simulink model "fusionAlg"  (R2018b)
settings: Solver=FixedStepDiscrete  StartTime=0.0  StopTime=inf  FixedStep=0.01  RelTol=1e-3
PostLoadFcn:
  | if any(exist('dsrtsu_mdlpostloadfcn', 'file') ~= 0), dsrtsu_mdlpostloadfcn('Execute', bdroot); end
model workspace (MAT data in the model file):
  handle : class17 (value not decoded)
(part 22 of 24)

== system fusionAlg/FUSION /FUS_DataAdapter/VisionAdapter/ObjAdapter/Obj_31/Subsystem ==
  <OBJ_Lat_Distance> : Inport
  <OBJ_Lat_Distance_STD> : Inport  Port=2
  <OBJ_Long_Distance> : Inport  Port=3
  <OBJ_Long_Distance_STD> : Inport  Port=4
  Bus Creator : BusCreator  Inputs=4  OutDataTypeStr=Bus: FUS_VISION_OBJ_COORD_ST
      settings: InheritFromInputs=off
  Obj_01_coordinate : Outport
  wires:
  <OBJ_Long_Distance>/1 -> Bus Creator/3
  <OBJ_Lat_Distance>/1 -> Bus Creator/1
  <OBJ_Lat_Distance_STD>/1 -> Bus Creator/2
  Bus Creator/1 -> Obj_01_coordinate/1
  <OBJ_Long_Distance_STD>/1 -> Bus Creator/4

== system fusionAlg/FUSION /FUS_DataAdapter/VisionAdapter/ObjAdapter/Obj_31/Subsystem1 ==
  <OBJ_Abs_Long_Velocity> : Inport
  <OBJ_Abs_Long_Velocity_STD> : Inport  Port=2
  <OBJ_Abs_Lat_Velocity> : Inport  Port=3
  <OBJ_Abs_Lat_Velocity_STD> : Inport  Port=4
  Bus Creator : BusCreator  Inputs=4  OutDataTypeStr=Bus: FUS_VISION_OBJ_VELOCITY
      settings: InheritFromInputs=off
  Out1 : Outport
  wires:
  <OBJ_Abs_Lat_Velocity_STD>/1 -> Bus Creator/4
  <OBJ_Abs_Long_Velocity>/1 -> Bus Creator/1
  <OBJ_Abs_Lat_Velocity>/1 -> Bus Creator/3
  <OBJ_Abs_Long_Velocity_STD>/1 -> Bus Creator/2
  Bus Creator/1 -> Out1/1

== system fusionAlg/FUSION /FUS_DataAdapter/VisionAdapter/ObjAdapter/Obj_31/Subsystem2 ==
  <OBJ_Angle_Mid> : Inport
  <OBJ_Angle_Mid_STD> : Inport  Port=2
  Bus Creator : BusCreator  Inputs=2  OutDataTypeStr=Bus: FUS_VISION_OBJ_ANGLE_ST
      settings: InheritFromInputs=off
  Out1 : Outport
  wires:
  <OBJ_Angle_Mid>/1 -> Bus Creator/1
  Bus Creator/1 -> Out1/1
  <OBJ_Angle_Mid_STD>/1 -> Bus Creator/2

== system fusionAlg/FUSION /FUS_DataAdapter/VisionAdapter/ObjAdapter/Obj_31/Subsystem3 ==
  <OBJ_Abs_Long_Acc> : Inport
  <OBJ_Abs_Long_Acc_STD> : Inport  Port=2
  <OBJ_Abs_Lat_Acc> : Inport  Port=3
  <OBJ_Abs_Lat_Acc_STD> : Inport  Port=4
  Bus Creator : BusCreator  Inputs=4  OutDataTypeStr=Bus: FUS_VISION_OBJ_ACCE_ST
      settings: InheritFromInputs=off
  Out1 : Outport
  wires:
  <OBJ_Abs_Long_Acc_STD>/1 -> Bus Creator/2
  <OBJ_Abs_Long_Acc>/1 -> Bus Creator/1
  Bus Creator/1 -> Out1/1
  <OBJ_Abs_Lat_Acc_STD>/1 -> Bus Creator/4
  <OBJ_Abs_Lat_Acc>/1 -> Bus Creator/3

== system fusionAlg/FUSION /FUS_DataAdapter/VisionAdapter/ObjAdapter/Obj_31/Subsystem4 ==
  <OBJ_Length> : Inport
  <OBJ_Width> : Inport  Port=2
  <OBJ_Height> : Inport  Port=3
  Bus Creator : BusCreator  Inputs=3  OutDataTypeStr=Bus: FUS_VISION_BOXSIZE_ST
      settings: InheritFromInputs=off
  Out1 : Outport
  wires:
  Bus Creator/1 -> Out1/1
  <OBJ_Height>/1 -> Bus Creator/3
  <OBJ_Width>/1 -> Bus Creator/2
  <OBJ_Length>/1 -> Bus Creator/1

== system fusionAlg/FUSION /FUS_DataAdapter/VisionAdapter/ObjAdapter/Obj_31/Subsystem5 ==
  Bus Creator : BusCreator  Inputs=3  OutDataTypeStr=Bus: FUS_VISOBJ_UINT8_RESERVED_ST
      settings: InheritFromInputs=off
  Constant1 : Constant  Value=0  OutDataTypeStr=uint8
  Constant2 : Constant  Value=0  OutDataTypeStr=uint8
  Constant3 : Constant  Value=0  OutDataTypeStr=uint8
  reserved1 : Outport
  wires:
  Bus Creator/1 -> reserved1/1
  Constant2/1 -> Bus Creator/1
  Constant1/1 -> Bus Creator/2
  Constant3/1 -> Bus Creator/3

== system fusionAlg/FUSION /FUS_DataAdapter/VisionAdapter/ObjAdapter/Obj_31/Subsystem6 ==
  Bus Creator : BusCreator  Inputs=2  OutDataTypeStr=Bus: FUS_VISOBJ_UINT32_RESERVED_ST
      settings: InheritFromInputs=off
  Constant5 : Constant  Value=0  OutDataTypeStr=uint32
  Constant6 : Constant  Value=0  OutDataTypeStr=uint32
  reserved2 : Outport
  wires:
  Constant5/1 -> Bus Creator/1
  Bus Creator/1 -> reserved2/1
  Constant6/1 -> Bus Creator/2

== system fusionAlg/FUSION /FUS_DataAdapter/VisionAdapter/ObjAdapter/Obj_31/Subsystem7 ==
  note: Fusion
  note: 0 : (BIT_0)Old or New
  note: EyeQ4
  note: 1 : (BIT_1)Predicted or Measured
  note: 2 : (BIT_2)Not Valid or Valid
  note: 0 : Initialized
  note: 1 : Measured
  note: 2 : Predicted
  <OBJ_Measuring_Status> : Inport
  1-D Lookup Table : Lookup_n-D  NumberOfTableDimensions=1  BreakpointsForDimension1=[0,1,2,3,4,5,6,7]  IndexSearchMethod=Linear search  Table=[2,0,1,1,0,0,1,1]  InterpMethod=Flat  InternalRulePriority=Speed  RndMeth=Simplest  InputSameDT=on
  Data Type Conversion1 : DataTypeConversion  OutDataTypeStr=uint32
  Obj_Status : Outport
  wires:
  Data Type Conversion1/1 -> Obj_Status/1  "Obj_Status"
  <OBJ_Measuring_Status>/1 -> 1-D Lookup Table/1
  1-D Lookup Table/1 -> Data Type Conversion1/1  "Obj_Status"

== system fusionAlg/FUSION /FUS_DataAdapter/VisionAdapter/ObjAdapter/Obj_31/Subsystem8 ==
  note: 2 : Truck
  note: 1 : Pedestrian
  note: 2 : Vehicle
  note: 0 : Unfilled
  note: EyeQ4
  note: Fusion
  note: 0 : Unknown
  note: 1 : CAR
  note: 3 : Motorbike
  note: 4 : Bicycle
  note: 5 : Pedestrian
  note: 6 : General_Object
  note: 7 : Animal
  note: 8 : Uncertain_Vcl
  note: 3 : Truck
  note: 4: MoTor bike
  note: 5 : Bicycle
  note: 6 : General object
  note: 7 : Animal
  <OBJ_Object_Class> : Inport
  1-D Lookup Table : Lookup_n-D  NumberOfTableDimensions=1  BreakpointsForDimension1=[0,1,2,3,4,5,6,7,8]  IndexSearchMethod=Linear search  Table=[0,2,3,4,5,1,6,7,0]  InterpMethod=Flat  InternalRulePriority=Speed  RndMeth=Simplest  InputSameDT=on
  Data Type Conversion2 : DataTypeConversion  OutDataTypeStr=uint32
  Obj_Type : Outport
  wires:
  1-D Lookup Table/1 -> Data Type Conversion2/1  "Obj_Status"
  <OBJ_Object_Class>/1 -> 1-D Lookup Table/1
  Data Type Conversion2/1 -> Obj_Type/1  "Obj_Type"

== system fusionAlg/FUSION /FUS_DataAdapter/VisionAdapter/ObjAdapter/Obj_32/Obj_01_Agge ==
  <OBJ_Object_Age> : Inport
  Bus Creator : BusCreator  Inputs=4  OutDataTypeStr=Bus: FUS_VISION_OBJ_STAGE_AGE_ST
      settings: InheritFromInputs=off
  Constant : Constant  Value=3  OutDataTypeStr=uint16
  Constant1 : Constant  Value=2  OutDataTypeStr=uint16
  Data Type Conversion : DataTypeConversion  OutDataTypeStr=uint16
  Obj_01_Age : Outport  OutDataTypeStr=Bus: FUS_VISION_OBJ_STAGE_AGE_ST
  wires:
  Bus Creator/1 -> Obj_01_Age/1
  Constant/1 -> Bus Creator/2
  <OBJ_Object_Age>/1 -> Data Type Conversion/1
  Constant1/1 -> Bus Creator/4
  Data Type Conversion/1 -> Bus Creator/3, Bus Creator/1  "measureAge"

== system fusionAlg/FUSION /FUS_DataAdapter/VisionAdapter/ObjAdapter/Obj_32/Obj_01_boundarhy ==
  Bus Creator : BusCreator  Inputs=4  OutDataTypeStr=Bus: FUS_VISION_OBJ_BOUNDARY
      settings: InheritFromInputs=off
  Constant{,1..3} (4 alike) : Constant  Value=0  OutDataTypeStr=int16
  Obj_01_boundary : Outport  OutDataTypeStr=Bus: FUS_VISION_OBJ_BOUNDARY
  wires:
  Bus Creator/1 -> Obj_01_boundary/1
  Constant/1 -> Bus Creator/1
  Constant1/1 -> Bus Creator/2
  Constant2/1 -> Bus Creator/3
  Constant3/1 -> Bus Creator/4

== system fusionAlg/FUSION /FUS_DataAdapter/VisionAdapter/ObjAdapter/Obj_32/Subsystem ==
  <OBJ_Lat_Distance> : Inport
  <OBJ_Lat_Distance_STD> : Inport  Port=2
  <OBJ_Long_Distance> : Inport  Port=3
  <OBJ_Long_Distance_STD> : Inport  Port=4
  Bus Creator : BusCreator  Inputs=4  OutDataTypeStr=Bus: FUS_VISION_OBJ_COORD_ST
      settings: InheritFromInputs=off
  Obj_01_coordinate : Outport
  wires:
  <OBJ_Long_Distance>/1 -> Bus Creator/3
  <OBJ_Lat_Distance>/1 -> Bus Creator/1
  <OBJ_Lat_Distance_STD>/1 -> Bus Creator/2
  Bus Creator/1 -> Obj_01_coordinate/1
  <OBJ_Long_Distance_STD>/1 -> Bus Creator/4

== system fusionAlg/FUSION /FUS_DataAdapter/VisionAdapter/ObjAdapter/Obj_32/Subsystem1 ==
  <OBJ_Abs_Long_Velocity> : Inport
  <OBJ_Abs_Long_Velocity_STD> : Inport  Port=2
  <OBJ_Abs_Lat_Velocity> : Inport  Port=3
  <OBJ_Abs_Lat_Velocity_STD> : Inport  Port=4
  Bus Creator : BusCreator  Inputs=4  OutDataTypeStr=Bus: FUS_VISION_OBJ_VELOCITY
      settings: InheritFromInputs=off
  Out1 : Outport
  wires:
  <OBJ_Abs_Lat_Velocity_STD>/1 -> Bus Creator/4
  <OBJ_Abs_Long_Velocity>/1 -> Bus Creator/1
  <OBJ_Abs_Lat_Velocity>/1 -> Bus Creator/3
  <OBJ_Abs_Long_Velocity_STD>/1 -> Bus Creator/2
  Bus Creator/1 -> Out1/1

== system fusionAlg/FUSION /FUS_DataAdapter/VisionAdapter/ObjAdapter/Obj_32/Subsystem2 ==
  <OBJ_Angle_Mid> : Inport
  <OBJ_Angle_Mid_STD> : Inport  Port=2
  Bus Creator : BusCreator  Inputs=2  OutDataTypeStr=Bus: FUS_VISION_OBJ_ANGLE_ST
      settings: InheritFromInputs=off
  Out1 : Outport
  wires:
  <OBJ_Angle_Mid>/1 -> Bus Creator/1
  Bus Creator/1 -> Out1/1
  <OBJ_Angle_Mid_STD>/1 -> Bus Creator/2

== system fusionAlg/FUSION /FUS_DataAdapter/VisionAdapter/ObjAdapter/Obj_32/Subsystem3 ==
  <OBJ_Abs_Long_Acc> : Inport
  <OBJ_Abs_Long_Acc_STD> : Inport  Port=2
  <OBJ_Abs_Lat_Acc> : Inport  Port=3
  <OBJ_Abs_Lat_Acc_STD> : Inport  Port=4
  Bus Creator : BusCreator  Inputs=4  OutDataTypeStr=Bus: FUS_VISION_OBJ_ACCE_ST
      settings: InheritFromInputs=off
  Out1 : Outport
  wires:
  <OBJ_Abs_Long_Acc_STD>/1 -> Bus Creator/2
  <OBJ_Abs_Long_Acc>/1 -> Bus Creator/1
  Bus Creator/1 -> Out1/1
  <OBJ_Abs_Lat_Acc_STD>/1 -> Bus Creator/4
  <OBJ_Abs_Lat_Acc>/1 -> Bus Creator/3

== system fusionAlg/FUSION /FUS_DataAdapter/VisionAdapter/ObjAdapter/Obj_32/Subsystem4 ==
  <OBJ_Length> : Inport
  <OBJ_Width> : Inport  Port=2
  <OBJ_Height> : Inport  Port=3
  Bus Creator : BusCreator  Inputs=3  OutDataTypeStr=Bus: FUS_VISION_BOXSIZE_ST
      settings: InheritFromInputs=off
  Out1 : Outport
  wires:
  Bus Creator/1 -> Out1/1
  <OBJ_Height>/1 -> Bus Creator/3
  <OBJ_Width>/1 -> Bus Creator/2
  <OBJ_Length>/1 -> Bus Creator/1

== system fusionAlg/FUSION /FUS_DataAdapter/VisionAdapter/ObjAdapter/Obj_32/Subsystem5 ==
  Bus Creator : BusCreator  Inputs=3  OutDataTypeStr=Bus: FUS_VISOBJ_UINT8_RESERVED_ST
      settings: InheritFromInputs=off
  Constant1 : Constant  Value=0  OutDataTypeStr=uint8
  Constant2 : Constant  Value=0  OutDataTypeStr=uint8
  Constant3 : Constant  Value=0  OutDataTypeStr=uint8
  reserved1 : Outport
  wires:
  Bus Creator/1 -> reserved1/1
  Constant2/1 -> Bus Creator/1
  Constant1/1 -> Bus Creator/2
  Constant3/1 -> Bus Creator/3

== system fusionAlg/FUSION /FUS_DataAdapter/VisionAdapter/ObjAdapter/Obj_32/Subsystem6 ==
  Bus Creator : BusCreator  Inputs=2  OutDataTypeStr=Bus: FUS_VISOBJ_UINT32_RESERVED_ST
      settings: InheritFromInputs=off
  Constant5 : Constant  Value=0  OutDataTypeStr=uint32
  Constant6 : Constant  Value=0  OutDataTypeStr=uint32
  reserved2 : Outport
  wires:
  Constant5/1 -> Bus Creator/1
  Bus Creator/1 -> reserved2/1
  Constant6/1 -> Bus Creator/2

== system fusionAlg/FUSION /FUS_DataAdapter/VisionAdapter/ObjAdapter/Obj_32/Subsystem7 ==
  note: Fusion
  note: 0 : (BIT_0)Old or New
  note: EyeQ4
  note: 1 : (BIT_1)Predicted or Measured
  note: 2 : (BIT_2)Not Valid or Valid
  note: 0 : Initialized
  note: 1 : Measured
  note: 2 : Predicted
  <OBJ_Measuring_Status> : Inport
  1-D Lookup Table : Lookup_n-D  NumberOfTableDimensions=1  BreakpointsForDimension1=[0,1,2,3,4,5,6,7]  IndexSearchMethod=Linear search  Table=[2,0,1,1,0,0,1,1]  InterpMethod=Flat  InternalRulePriority=Speed  RndMeth=Simplest  InputSameDT=on
  Data Type Conversion1 : DataTypeConversion  OutDataTypeStr=uint32
  Obj_Status : Outport
  wires:
  Data Type Conversion1/1 -> Obj_Status/1  "Obj_Status"
  <OBJ_Measuring_Status>/1 -> 1-D Lookup Table/1
  1-D Lookup Table/1 -> Data Type Conversion1/1  "Obj_Status"

== system fusionAlg/FUSION /FUS_DataAdapter/VisionAdapter/ObjAdapter/Obj_32/Subsystem8 ==
  note: 2 : Truck
  note: 1 : Pedestrian
  note: 2 : Vehicle
  note: 0 : Unfilled
  note: EyeQ4
  note: Fusion
  note: 0 : Unknown
  note: 1 : CAR
  note: 3 : Motorbike
  note: 4 : Bicycle
  note: 5 : Pedestrian
  note: 6 : General_Object
  note: 7 : Animal
  note: 8 : Uncertain_Vcl
  note: 3 : Truck
  note: 4: MoTor bike
  note: 5 : Bicycle
  note: 6 : General object
  note: 7 : Animal
  <OBJ_Object_Class> : Inport
  1-D Lookup Table : Lookup_n-D  NumberOfTableDimensions=1  BreakpointsForDimension1=[0,1,2,3,4,5,6,7,8]  IndexSearchMethod=Linear search  Table=[0,2,3,4,5,1,6,7,0]  InterpMethod=Flat  InternalRulePriority=Speed  RndMeth=Simplest  InputSameDT=on
  Data Type Conversion2 : DataTypeConversion  OutDataTypeStr=uint32
  Obj_Type : Outport
  wires:
  1-D Lookup Table/1 -> Data Type Conversion2/1  "Obj_Status"
  <OBJ_Object_Class>/1 -> 1-D Lookup Table/1
  Data Type Conversion2/1 -> Obj_Type/1  "Obj_Type"

== system fusionAlg/FUSION /FUS_DataAdapter/VisionAdapter/ObjAdapter/Obj_33/Obj_01_Agge ==
  <OBJ_Object_Age> : Inport
  Bus Creator : BusCreator  Inputs=4  OutDataTypeStr=Bus: FUS_VISION_OBJ_STAGE_AGE_ST
      settings: InheritFromInputs=off
  Constant : Constant  Value=3  OutDataTypeStr=uint16
  Constant1 : Constant  Value=2  OutDataTypeStr=uint16
  Data Type Conversion : DataTypeConversion  OutDataTypeStr=uint16
  Obj_01_Age : Outport  OutDataTypeStr=Bus: FUS_VISION_OBJ_STAGE_AGE_ST
  wires:
  Bus Creator/1 -> Obj_01_Age/1
  Constant/1 -> Bus Creator/2
  <OBJ_Object_Age>/1 -> Data Type Conversion/1
  Constant1/1 -> Bus Creator/4
  Data Type Conversion/1 -> Bus Creator/3, Bus Creator/1  "measureAge"

== system fusionAlg/FUSION /FUS_DataAdapter/VisionAdapter/ObjAdapter/Obj_33/Obj_01_boundarhy ==
  Bus Creator : BusCreator  Inputs=4  OutDataTypeStr=Bus: FUS_VISION_OBJ_BOUNDARY
      settings: InheritFromInputs=off
  Constant{,1..3} (4 alike) : Constant  Value=0  OutDataTypeStr=int16
  Obj_01_boundary : Outport  OutDataTypeStr=Bus: FUS_VISION_OBJ_BOUNDARY
  wires:
  Bus Creator/1 -> Obj_01_boundary/1
  Constant/1 -> Bus Creator/1
  Constant1/1 -> Bus Creator/2
  Constant2/1 -> Bus Creator/3
  Constant3/1 -> Bus Creator/4

== system fusionAlg/FUSION /FUS_DataAdapter/VisionAdapter/ObjAdapter/Obj_33/Subsystem ==
  <OBJ_Lat_Distance> : Inport
  <OBJ_Lat_Distance_STD> : Inport  Port=2
  <OBJ_Long_Distance> : Inport  Port=3
  <OBJ_Long_Distance_STD> : Inport  Port=4
  Bus Creator : BusCreator  Inputs=4  OutDataTypeStr=Bus: FUS_VISION_OBJ_COORD_ST
      settings: InheritFromInputs=off
  Obj_01_coordinate : Outport
  wires:
  <OBJ_Long_Distance>/1 -> Bus Creator/3
  <OBJ_Lat_Distance>/1 -> Bus Creator/1
  <OBJ_Lat_Distance_STD>/1 -> Bus Creator/2
  Bus Creator/1 -> Obj_01_coordinate/1
  <OBJ_Long_Distance_STD>/1 -> Bus Creator/4

== system fusionAlg/FUSION /FUS_DataAdapter/VisionAdapter/ObjAdapter/Obj_33/Subsystem1 ==
  <OBJ_Abs_Long_Velocity> : Inport
  <OBJ_Abs_Long_Velocity_STD> : Inport  Port=2
  <OBJ_Abs_Lat_Velocity> : Inport  Port=3
  <OBJ_Abs_Lat_Velocity_STD> : Inport  Port=4
  Bus Creator : BusCreator  Inputs=4  OutDataTypeStr=Bus: FUS_VISION_OBJ_VELOCITY
      settings: InheritFromInputs=off
  Out1 : Outport
  wires:
  <OBJ_Abs_Lat_Velocity_STD>/1 -> Bus Creator/4
  <OBJ_Abs_Long_Velocity>/1 -> Bus Creator/1
  <OBJ_Abs_Lat_Velocity>/1 -> Bus Creator/3
  <OBJ_Abs_Long_Velocity_STD>/1 -> Bus Creator/2
  Bus Creator/1 -> Out1/1

== system fusionAlg/FUSION /FUS_DataAdapter/VisionAdapter/ObjAdapter/Obj_33/Subsystem2 ==
  <OBJ_Angle_Mid> : Inport
  <OBJ_Angle_Mid_STD> : Inport  Port=2
  Bus Creator : BusCreator  Inputs=2  OutDataTypeStr=Bus: FUS_VISION_OBJ_ANGLE_ST
      settings: InheritFromInputs=off
  Out1 : Outport
  wires:
  <OBJ_Angle_Mid>/1 -> Bus Creator/1
  Bus Creator/1 -> Out1/1
  <OBJ_Angle_Mid_STD>/1 -> Bus Creator/2

== system fusionAlg/FUSION /FUS_DataAdapter/VisionAdapter/ObjAdapter/Obj_33/Subsystem3 ==
  <OBJ_Abs_Long_Acc> : Inport
  <OBJ_Abs_Long_Acc_STD> : Inport  Port=2
  <OBJ_Abs_Lat_Acc> : Inport  Port=3
  <OBJ_Abs_Lat_Acc_STD> : Inport  Port=4
  Bus Creator : BusCreator  Inputs=4  OutDataTypeStr=Bus: FUS_VISION_OBJ_ACCE_ST
      settings: InheritFromInputs=off
  Out1 : Outport
  wires:
  <OBJ_Abs_Long_Acc_STD>/1 -> Bus Creator/2
  <OBJ_Abs_Long_Acc>/1 -> Bus Creator/1
  Bus Creator/1 -> Out1/1
  <OBJ_Abs_Lat_Acc_STD>/1 -> Bus Creator/4
  <OBJ_Abs_Lat_Acc>/1 -> Bus Creator/3

== system fusionAlg/FUSION /FUS_DataAdapter/VisionAdapter/ObjAdapter/Obj_33/Subsystem4 ==
  <OBJ_Length> : Inport
  <OBJ_Width> : Inport  Port=2
  <OBJ_Height> : Inport  Port=3
  Bus Creator : BusCreator  Inputs=3  OutDataTypeStr=Bus: FUS_VISION_BOXSIZE_ST
      settings: InheritFromInputs=off
  Out1 : Outport
  wires:
  Bus Creator/1 -> Out1/1
  <OBJ_Height>/1 -> Bus Creator/3
  <OBJ_Width>/1 -> Bus Creator/2
  <OBJ_Length>/1 -> Bus Creator/1

== system fusionAlg/FUSION /FUS_DataAdapter/VisionAdapter/ObjAdapter/Obj_33/Subsystem5 ==
  Bus Creator : BusCreator  Inputs=3  OutDataTypeStr=Bus: FUS_VISOBJ_UINT8_RESERVED_ST
      settings: InheritFromInputs=off
  Constant1 : Constant  Value=0  OutDataTypeStr=uint8
  Constant2 : Constant  Value=0  OutDataTypeStr=uint8
  Constant3 : Constant  Value=0  OutDataTypeStr=uint8
  reserved1 : Outport
  wires:
  Bus Creator/1 -> reserved1/1
  Constant2/1 -> Bus Creator/1
  Constant1/1 -> Bus Creator/2
  Constant3/1 -> Bus Creator/3

== system fusionAlg/FUSION /FUS_DataAdapter/VisionAdapter/ObjAdapter/Obj_33/Subsystem6 ==
  Bus Creator : BusCreator  Inputs=2  OutDataTypeStr=Bus: FUS_VISOBJ_UINT32_RESERVED_ST
      settings: InheritFromInputs=off
  Constant5 : Constant  Value=0  OutDataTypeStr=uint32
  Constant6 : Constant  Value=0  OutDataTypeStr=uint32
  reserved2 : Outport
  wires:
  Constant5/1 -> Bus Creator/1
  Bus Creator/1 -> reserved2/1
  Constant6/1 -> Bus Creator/2

== system fusionAlg/FUSION /FUS_DataAdapter/VisionAdapter/ObjAdapter/Obj_33/Subsystem7 ==
  note: Fusion
  note: 0 : (BIT_0)Old or New
  note: EyeQ4
  note: 1 : (BIT_1)Predicted or Measured
  note: 2 : (BIT_2)Not Valid or Valid
  note: 0 : Initialized
  note: 1 : Measured
  note: 2 : Predicted
  <OBJ_Measuring_Status> : Inport
  1-D Lookup Table : Lookup_n-D  NumberOfTableDimensions=1  BreakpointsForDimension1=[0,1,2,3,4,5,6,7]  IndexSearchMethod=Linear search  Table=[2,0,1,1,0,0,1,1]  InterpMethod=Flat  InternalRulePriority=Speed  RndMeth=Simplest  InputSameDT=on
  Data Type Conversion1 : DataTypeConversion  OutDataTypeStr=uint32
  Obj_Status : Outport
  wires:
  Data Type Conversion1/1 -> Obj_Status/1  "Obj_Status"
  <OBJ_Measuring_Status>/1 -> 1-D Lookup Table/1
  1-D Lookup Table/1 -> Data Type Conversion1/1  "Obj_Status"

== system fusionAlg/FUSION /FUS_DataAdapter/VisionAdapter/ObjAdapter/Obj_33/Subsystem8 ==
  note: 2 : Truck
  note: 1 : Pedestrian
  note: 2 : Vehicle
  note: 0 : Unfilled
  note: EyeQ4
  note: Fusion
  note: 0 : Unknown
  note: 1 : CAR
  note: 3 : Motorbike
  note: 4 : Bicycle
  note: 5 : Pedestrian
  note: 6 : General_Object
  note: 7 : Animal
  note: 8 : Uncertain_Vcl
  note: 3 : Truck
  note: 4: MoTor bike
  note: 5 : Bicycle
  note: 6 : General object
  note: 7 : Animal
  <OBJ_Object_Class> : Inport
  1-D Lookup Table : Lookup_n-D  NumberOfTableDimensions=1  BreakpointsForDimension1=[0,1,2,3,4,5,6,7,8]  IndexSearchMethod=Linear search  Table=[0,2,3,4,5,1,6,7,0]  InterpMethod=Flat  InternalRulePriority=Speed  RndMeth=Simplest  InputSameDT=on
  Data Type Conversion2 : DataTypeConversion  OutDataTypeStr=uint32
  Obj_Type : Outport
  wires:
  1-D Lookup Table/1 -> Data Type Conversion2/1  "Obj_Status"
  <OBJ_Object_Class>/1 -> 1-D Lookup Table/1
  Data Type Conversion2/1 -> Obj_Type/1  "Obj_Type"

== system fusionAlg/FUSION /FUS_DataAdapter/VisionAdapter/ObjAdapter/Obj_34/Obj_01_Agge ==
  <OBJ_Object_Age> : Inport
  Bus Creator : BusCreator  Inputs=4  OutDataTypeStr=Bus: FUS_VISION_OBJ_STAGE_AGE_ST
      settings: InheritFromInputs=off
  Constant : Constant  Value=3  OutDataTypeStr=uint16
  Constant1 : Constant  Value=2  OutDataTypeStr=uint16
  Data Type Conversion : DataTypeConversion  OutDataTypeStr=uint16
  Obj_01_Age : Outport  OutDataTypeStr=Bus: FUS_VISION_OBJ_STAGE_AGE_ST
  wires:
  Bus Creator/1 -> Obj_01_Age/1
  Constant/1 -> Bus Creator/2
  <OBJ_Object_Age>/1 -> Data Type Conversion/1
  Constant1/1 -> Bus Creator/4
  Data Type Conversion/1 -> Bus Creator/3, Bus Creator/1  "measureAge"

== system fusionAlg/FUSION /FUS_DataAdapter/VisionAdapter/ObjAdapter/Obj_34/Obj_01_boundarhy ==
  Bus Creator : BusCreator  Inputs=4  OutDataTypeStr=Bus: FUS_VISION_OBJ_BOUNDARY
      settings: InheritFromInputs=off
  Constant{,1..3} (4 alike) : Constant  Value=0  OutDataTypeStr=int16
  Obj_01_boundary : Outport  OutDataTypeStr=Bus: FUS_VISION_OBJ_BOUNDARY
  wires:
  Bus Creator/1 -> Obj_01_boundary/1
  Constant/1 -> Bus Creator/1
  Constant1/1 -> Bus Creator/2
  Constant2/1 -> Bus Creator/3
  Constant3/1 -> Bus Creator/4

== system fusionAlg/FUSION /FUS_DataAdapter/VisionAdapter/ObjAdapter/Obj_34/Subsystem ==
  <OBJ_Lat_Distance> : Inport
  <OBJ_Lat_Distance_STD> : Inport  Port=2
  <OBJ_Long_Distance> : Inport  Port=3
  <OBJ_Long_Distance_STD> : Inport  Port=4
  Bus Creator : BusCreator  Inputs=4  OutDataTypeStr=Bus: FUS_VISION_OBJ_COORD_ST
      settings: InheritFromInputs=off
  Obj_01_coordinate : Outport
  wires:
  <OBJ_Long_Distance>/1 -> Bus Creator/3
  <OBJ_Lat_Distance>/1 -> Bus Creator/1
  <OBJ_Lat_Distance_STD>/1 -> Bus Creator/2
  Bus Creator/1 -> Obj_01_coordinate/1
  <OBJ_Long_Distance_STD>/1 -> Bus Creator/4

== system fusionAlg/FUSION /FUS_DataAdapter/VisionAdapter/ObjAdapter/Obj_34/Subsystem1 ==
  <OBJ_Abs_Long_Velocity> : Inport
  <OBJ_Abs_Long_Velocity_STD> : Inport  Port=2
  <OBJ_Abs_Lat_Velocity> : Inport  Port=3
  <OBJ_Abs_Lat_Velocity_STD> : Inport  Port=4
  Bus Creator : BusCreator  Inputs=4  OutDataTypeStr=Bus: FUS_VISION_OBJ_VELOCITY
      settings: InheritFromInputs=off
  Out1 : Outport
  wires:
  <OBJ_Abs_Lat_Velocity_STD>/1 -> Bus Creator/4
  <OBJ_Abs_Long_Velocity>/1 -> Bus Creator/1
  <OBJ_Abs_Lat_Velocity>/1 -> Bus Creator/3
  <OBJ_Abs_Long_Velocity_STD>/1 -> Bus Creator/2
  Bus Creator/1 -> Out1/1

== system fusionAlg/FUSION /FUS_DataAdapter/VisionAdapter/ObjAdapter/Obj_34/Subsystem2 ==
  <OBJ_Angle_Mid> : Inport
  <OBJ_Angle_Mid_STD> : Inport  Port=2
  Bus Creator : BusCreator  Inputs=2  OutDataTypeStr=Bus: FUS_VISION_OBJ_ANGLE_ST
      settings: InheritFromInputs=off
  Out1 : Outport
  wires:
  <OBJ_Angle_Mid>/1 -> Bus Creator/1
  Bus Creator/1 -> Out1/1
  <OBJ_Angle_Mid_STD>/1 -> Bus Creator/2

== system fusionAlg/FUSION /FUS_DataAdapter/VisionAdapter/ObjAdapter/Obj_34/Subsystem3 ==
  <OBJ_Abs_Long_Acc> : Inport
  <OBJ_Abs_Long_Acc_STD> : Inport  Port=2
  <OBJ_Abs_Lat_Acc> : Inport  Port=3
  <OBJ_Abs_Lat_Acc_STD> : Inport  Port=4
  Bus Creator : BusCreator  Inputs=4  OutDataTypeStr=Bus: FUS_VISION_OBJ_ACCE_ST
      settings: InheritFromInputs=off
  Out1 : Outport
  wires:
  <OBJ_Abs_Long_Acc_STD>/1 -> Bus Creator/2
  <OBJ_Abs_Long_Acc>/1 -> Bus Creator/1
  Bus Creator/1 -> Out1/1
  <OBJ_Abs_Lat_Acc_STD>/1 -> Bus Creator/4
  <OBJ_Abs_Lat_Acc>/1 -> Bus Creator/3

== system fusionAlg/FUSION /FUS_DataAdapter/VisionAdapter/ObjAdapter/Obj_34/Subsystem4 ==
  <OBJ_Length> : Inport
  <OBJ_Width> : Inport  Port=2
  <OBJ_Height> : Inport  Port=3
  Bus Creator : BusCreator  Inputs=3  OutDataTypeStr=Bus: FUS_VISION_BOXSIZE_ST
      settings: InheritFromInputs=off
  Out1 : Outport
  wires:
  Bus Creator/1 -> Out1/1
  <OBJ_Height>/1 -> Bus Creator/3
  <OBJ_Width>/1 -> Bus Creator/2
  <OBJ_Length>/1 -> Bus Creator/1

== system fusionAlg/FUSION /FUS_DataAdapter/VisionAdapter/ObjAdapter/Obj_34/Subsystem5 ==
  Bus Creator : BusCreator  Inputs=3  OutDataTypeStr=Bus: FUS_VISOBJ_UINT8_RESERVED_ST
      settings: InheritFromInputs=off
  Constant1 : Constant  Value=0  OutDataTypeStr=uint8
  Constant2 : Constant  Value=0  OutDataTypeStr=uint8
  Constant3 : Constant  Value=0  OutDataTypeStr=uint8
  reserved1 : Outport
  wires:
  Bus Creator/1 -> reserved1/1
  Constant2/1 -> Bus Creator/1
  Constant1/1 -> Bus Creator/2
  Constant3/1 -> Bus Creator/3

== system fusionAlg/FUSION /FUS_DataAdapter/VisionAdapter/ObjAdapter/Obj_34/Subsystem6 ==
  Bus Creator : BusCreator  Inputs=2  OutDataTypeStr=Bus: FUS_VISOBJ_UINT32_RESERVED_ST
      settings: InheritFromInputs=off
  Constant5 : Constant  Value=0  OutDataTypeStr=uint32
  Constant6 : Constant  Value=0  OutDataTypeStr=uint32
  reserved2 : Outport
  wires:
  Constant5/1 -> Bus Creator/1
  Bus Creator/1 -> reserved2/1
  Constant6/1 -> Bus Creator/2

== system fusionAlg/FUSION /FUS_DataAdapter/VisionAdapter/ObjAdapter/Obj_34/Subsystem7 ==
  note: Fusion
  note: 0 : (BIT_0)Old or New
  note: EyeQ4
  note: 1 : (BIT_1)Predicted or Measured
  note: 2 : (BIT_2)Not Valid or Valid
  note: 0 : Initialized
  note: 1 : Measured
  note: 2 : Predicted
  <OBJ_Measuring_Status> : Inport
  1-D Lookup Table : Lookup_n-D  NumberOfTableDimensions=1  BreakpointsForDimension1=[0,1,2,3,4,5,6,7]  IndexSearchMethod=Linear search  Table=[2,0,1,1,0,0,1,1]  InterpMethod=Flat  InternalRulePriority=Speed  RndMeth=Simplest  InputSameDT=on
  Data Type Conversion1 : DataTypeConversion  OutDataTypeStr=uint32
  Obj_Status : Outport
  wires:
  Data Type Conversion1/1 -> Obj_Status/1  "Obj_Status"
  <OBJ_Measuring_Status>/1 -> 1-D Lookup Table/1
  1-D Lookup Table/1 -> Data Type Conversion1/1  "Obj_Status"

== system fusionAlg/FUSION /FUS_DataAdapter/VisionAdapter/ObjAdapter/Obj_34/Subsystem8 ==
  note: 2 : Truck
  note: 1 : Pedestrian
  note: 2 : Vehicle
  note: 0 : Unfilled
  note: EyeQ4
  note: Fusion
  note: 0 : Unknown
  note: 1 : CAR
  note: 3 : Motorbike
  note: 4 : Bicycle
  note: 5 : Pedestrian
  note: 6 : General_Object
  note: 7 : Animal
  note: 8 : Uncertain_Vcl
  note: 3 : Truck
  note: 4: MoTor bike
  note: 5 : Bicycle
  note: 6 : General object
  note: 7 : Animal
  <OBJ_Object_Class> : Inport
  1-D Lookup Table : Lookup_n-D  NumberOfTableDimensions=1  BreakpointsForDimension1=[0,1,2,3,4,5,6,7,8]  IndexSearchMethod=Linear search  Table=[0,2,3,4,5,1,6,7,0]  InterpMethod=Flat  InternalRulePriority=Speed  RndMeth=Simplest  InputSameDT=on
  Data Type Conversion2 : DataTypeConversion  OutDataTypeStr=uint32
  Obj_Type : Outport
  wires:
  1-D Lookup Table/1 -> Data Type Conversion2/1  "Obj_Status"
  <OBJ_Object_Class>/1 -> 1-D Lookup Table/1
  Data Type Conversion2/1 -> Obj_Type/1  "Obj_Type"

== system fusionAlg/FUSION /FUS_DataAdapter/VisionAdapter/ObjAdapter/Obj_35/Obj_01_Agge ==
  <OBJ_Object_Age> : Inport
  Bus Creator : BusCreator  Inputs=4  OutDataTypeStr=Bus: FUS_VISION_OBJ_STAGE_AGE_ST
      settings: InheritFromInputs=off
  Constant : Constant  Value=3  OutDataTypeStr=uint16
  Constant1 : Constant  Value=2  OutDataTypeStr=uint16
  Data Type Conversion : DataTypeConversion  OutDataTypeStr=uint16
  Obj_01_Age : Outport  OutDataTypeStr=Bus: FUS_VISION_OBJ_STAGE_AGE_ST
  wires:
  Bus Creator/1 -> Obj_01_Age/1
  Constant/1 -> Bus Creator/2
  <OBJ_Object_Age>/1 -> Data Type Conversion/1
  Constant1/1 -> Bus Creator/4
  Data Type Conversion/1 -> Bus Creator/3, Bus Creator/1  "measureAge"

== system fusionAlg/FUSION /FUS_DataAdapter/VisionAdapter/ObjAdapter/Obj_35/Obj_01_boundarhy ==
  Bus Creator : BusCreator  Inputs=4  OutDataTypeStr=Bus: FUS_VISION_OBJ_BOUNDARY
      settings: InheritFromInputs=off
  Constant{,1..3} (4 alike) : Constant  Value=0  OutDataTypeStr=int16
  Obj_01_boundary : Outport  OutDataTypeStr=Bus: FUS_VISION_OBJ_BOUNDARY
  wires:
  Bus Creator/1 -> Obj_01_boundary/1
  Constant/1 -> Bus Creator/1
  Constant1/1 -> Bus Creator/2
  Constant2/1 -> Bus Creator/3
  Constant3/1 -> Bus Creator/4

== system fusionAlg/FUSION /FUS_DataAdapter/VisionAdapter/ObjAdapter/Obj_35/Subsystem ==
  <OBJ_Lat_Distance> : Inport
  <OBJ_Lat_Distance_STD> : Inport  Port=2
  <OBJ_Long_Distance> : Inport  Port=3
  <OBJ_Long_Distance_STD> : Inport  Port=4
  Bus Creator : BusCreator  Inputs=4  OutDataTypeStr=Bus: FUS_VISION_OBJ_COORD_ST
      settings: InheritFromInputs=off
  Obj_01_coordinate : Outport
  wires:
  <OBJ_Long_Distance>/1 -> Bus Creator/3
  <OBJ_Lat_Distance>/1 -> Bus Creator/1
  <OBJ_Lat_Distance_STD>/1 -> Bus Creator/2
  Bus Creator/1 -> Obj_01_coordinate/1
  <OBJ_Long_Distance_STD>/1 -> Bus Creator/4

== system fusionAlg/FUSION /FUS_DataAdapter/VisionAdapter/ObjAdapter/Obj_35/Subsystem1 ==
  <OBJ_Abs_Long_Velocity> : Inport
  <OBJ_Abs_Long_Velocity_STD> : Inport  Port=2
  <OBJ_Abs_Lat_Velocity> : Inport  Port=3
  <OBJ_Abs_Lat_Velocity_STD> : Inport  Port=4
  Bus Creator : BusCreator  Inputs=4  OutDataTypeStr=Bus: FUS_VISION_OBJ_VELOCITY
      settings: InheritFromInputs=off
  Out1 : Outport
  wires:
  <OBJ_Abs_Lat_Velocity_STD>/1 -> Bus Creator/4
  <OBJ_Abs_Long_Velocity>/1 -> Bus Creator/1
  <OBJ_Abs_Lat_Velocity>/1 -> Bus Creator/3
  <OBJ_Abs_Long_Velocity_STD>/1 -> Bus Creator/2
  Bus Creator/1 -> Out1/1

== system fusionAlg/FUSION /FUS_DataAdapter/VisionAdapter/ObjAdapter/Obj_35/Subsystem2 ==
  <OBJ_Angle_Mid> : Inport
  <OBJ_Angle_Mid_STD> : Inport  Port=2
  Bus Creator : BusCreator  Inputs=2  OutDataTypeStr=Bus: FUS_VISION_OBJ_ANGLE_ST
      settings: InheritFromInputs=off
  Out1 : Outport
  wires:
  <OBJ_Angle_Mid>/1 -> Bus Creator/1
  Bus Creator/1 -> Out1/1
  <OBJ_Angle_Mid_STD>/1 -> Bus Creator/2

== system fusionAlg/FUSION /FUS_DataAdapter/VisionAdapter/ObjAdapter/Obj_35/Subsystem3 ==
  <OBJ_Abs_Long_Acc> : Inport
  <OBJ_Abs_Long_Acc_STD> : Inport  Port=2
  <OBJ_Abs_Lat_Acc> : Inport  Port=3
  <OBJ_Abs_Lat_Acc_STD> : Inport  Port=4
  Bus Creator : BusCreator  Inputs=4  OutDataTypeStr=Bus: FUS_VISION_OBJ_ACCE_ST
      settings: InheritFromInputs=off
  Out1 : Outport
  wires:
  <OBJ_Abs_Long_Acc_STD>/1 -> Bus Creator/2
  <OBJ_Abs_Long_Acc>/1 -> Bus Creator/1
  Bus Creator/1 -> Out1/1
  <OBJ_Abs_Lat_Acc_STD>/1 -> Bus Creator/4
  <OBJ_Abs_Lat_Acc>/1 -> Bus Creator/3

== system fusionAlg/FUSION /FUS_DataAdapter/VisionAdapter/ObjAdapter/Obj_35/Subsystem4 ==
  <OBJ_Length> : Inport
  <OBJ_Width> : Inport  Port=2
  <OBJ_Height> : Inport  Port=3
  Bus Creator : BusCreator  Inputs=3  OutDataTypeStr=Bus: FUS_VISION_BOXSIZE_ST
      settings: InheritFromInputs=off
  Out1 : Outport
  wires:
  Bus Creator/1 -> Out1/1
  <OBJ_Height>/1 -> Bus Creator/3
  <OBJ_Width>/1 -> Bus Creator/2
  <OBJ_Length>/1 -> Bus Creator/1

== system fusionAlg/FUSION /FUS_DataAdapter/VisionAdapter/ObjAdapter/Obj_35/Subsystem5 ==
  Bus Creator : BusCreator  Inputs=3  OutDataTypeStr=Bus: FUS_VISOBJ_UINT8_RESERVED_ST
      settings: InheritFromInputs=off
  Constant1 : Constant  Value=0  OutDataTypeStr=uint8
  Constant2 : Constant  Value=0  OutDataTypeStr=uint8
  Constant3 : Constant  Value=0  OutDataTypeStr=uint8
  reserved1 : Outport
  wires:
  Bus Creator/1 -> reserved1/1
  Constant2/1 -> Bus Creator/1
  Constant1/1 -> Bus Creator/2
  Constant3/1 -> Bus Creator/3

== system fusionAlg/FUSION /FUS_DataAdapter/VisionAdapter/ObjAdapter/Obj_35/Subsystem6 ==
  Bus Creator : BusCreator  Inputs=2  OutDataTypeStr=Bus: FUS_VISOBJ_UINT32_RESERVED_ST
      settings: InheritFromInputs=off
  Constant5 : Constant  Value=0  OutDataTypeStr=uint32
  Constant6 : Constant  Value=0  OutDataTypeStr=uint32
  reserved2 : Outport
  wires:
  Constant5/1 -> Bus Creator/1
  Bus Creator/1 -> reserved2/1
  Constant6/1 -> Bus Creator/2

== system fusionAlg/FUSION /FUS_DataAdapter/VisionAdapter/ObjAdapter/Obj_35/Subsystem7 ==
  note: Fusion
  note: 0 : (BIT_0)Old or New
  note: EyeQ4
  note: 1 : (BIT_1)Predicted or Measured
  note: 2 : (BIT_2)Not Valid or Valid
  note: 0 : Initialized
  note: 1 : Measured
  note: 2 : Predicted
  <OBJ_Measuring_Status> : Inport
  1-D Lookup Table : Lookup_n-D  NumberOfTableDimensions=1  BreakpointsForDimension1=[0,1,2,3,4,5,6,7]  IndexSearchMethod=Linear search  Table=[2,0,1,1,0,0,1,1]  InterpMethod=Flat  InternalRulePriority=Speed  RndMeth=Simplest  InputSameDT=on
  Data Type Conversion1 : DataTypeConversion  OutDataTypeStr=uint32
  Obj_Status : Outport
  wires:
  Data Type Conversion1/1 -> Obj_Status/1  "Obj_Status"
  <OBJ_Measuring_Status>/1 -> 1-D Lookup Table/1
  1-D Lookup Table/1 -> Data Type Conversion1/1  "Obj_Status"

== system fusionAlg/FUSION /FUS_DataAdapter/VisionAdapter/ObjAdapter/Obj_35/Subsystem8 ==
  note: 2 : Truck
  note: 1 : Pedestrian
  note: 2 : Vehicle
  note: 0 : Unfilled
  note: EyeQ4
  note: Fusion
  note: 0 : Unknown
  note: 1 : CAR
  note: 3 : Motorbike
  note: 4 : Bicycle
  note: 5 : Pedestrian
  note: 6 : General_Object
  note: 7 : Animal
  note: 8 : Uncertain_Vcl
  note: 3 : Truck
  note: 4: MoTor bike
  note: 5 : Bicycle
  note: 6 : General object
  note: 7 : Animal
  <OBJ_Object_Class> : Inport
  1-D Lookup Table : Lookup_n-D  NumberOfTableDimensions=1  BreakpointsForDimension1=[0,1,2,3,4,5,6,7,8]  IndexSearchMethod=Linear search  Table=[0,2,3,4,5,1,6,7,0]  InterpMethod=Flat  InternalRulePriority=Speed  RndMeth=Simplest  InputSameDT=on
  Data Type Conversion2 : DataTypeConversion  OutDataTypeStr=uint32
  Obj_Type : Outport
  wires:
  1-D Lookup Table/1 -> Data Type Conversion2/1  "Obj_Status"
  <OBJ_Object_Class>/1 -> 1-D Lookup Table/1
  Data Type Conversion2/1 -> Obj_Type/1  "Obj_Type"

== system fusionAlg/FUSION /FUS_DataAdapter/VisionAdapter/ObjAdapter/Obj_36/Obj_01_Agge ==
  <OBJ_Object_Age> : Inport
  Bus Creator : BusCreator  Inputs=4  OutDataTypeStr=Bus: FUS_VISION_OBJ_STAGE_AGE_ST
      settings: InheritFromInputs=off
  Constant : Constant  Value=3  OutDataTypeStr=uint16
  Constant1 : Constant  Value=2  OutDataTypeStr=uint16
  Data Type Conversion : DataTypeConversion  OutDataTypeStr=uint16
  Obj_01_Age : Outport  OutDataTypeStr=Bus: FUS_VISION_OBJ_STAGE_AGE_ST
  wires:
  Bus Creator/1 -> Obj_01_Age/1
  Constant/1 -> Bus Creator/2
  <OBJ_Object_Age>/1 -> Data Type Conversion/1
  Constant1/1 -> Bus Creator/4
  Data Type Conversion/1 -> Bus Creator/3, Bus Creator/1  "measureAge"

== system fusionAlg/FUSION /FUS_DataAdapter/VisionAdapter/ObjAdapter/Obj_36/Obj_01_boundarhy ==
  Bus Creator : BusCreator  Inputs=4  OutDataTypeStr=Bus: FUS_VISION_OBJ_BOUNDARY
      settings: InheritFromInputs=off
  Constant{,1..3} (4 alike) : Constant  Value=0  OutDataTypeStr=int16
  Obj_01_boundary : Outport  OutDataTypeStr=Bus: FUS_VISION_OBJ_BOUNDARY
  wires:
  Bus Creator/1 -> Obj_01_boundary/1
  Constant/1 -> Bus Creator/1
  Constant1/1 -> Bus Creator/2
  Constant2/1 -> Bus Creator/3
  Constant3/1 -> Bus Creator/4

== system fusionAlg/FUSION /FUS_DataAdapter/VisionAdapter/ObjAdapter/Obj_36/Subsystem ==
  <OBJ_Lat_Distance> : Inport
  <OBJ_Lat_Distance_STD> : Inport  Port=2
  <OBJ_Long_Distance> : Inport  Port=3
  <OBJ_Long_Distance_STD> : Inport  Port=4
  Bus Creator : BusCreator  Inputs=4  OutDataTypeStr=Bus: FUS_VISION_OBJ_COORD_ST
      settings: InheritFromInputs=off
  Obj_01_coordinate : Outport
  wires:
  <OBJ_Long_Distance>/1 -> Bus Creator/3
  <OBJ_Lat_Distance>/1 -> Bus Creator/1
  <OBJ_Lat_Distance_STD>/1 -> Bus Creator/2
  Bus Creator/1 -> Obj_01_coordinate/1
  <OBJ_Long_Distance_STD>/1 -> Bus Creator/4

== system fusionAlg/FUSION /FUS_DataAdapter/VisionAdapter/ObjAdapter/Obj_36/Subsystem1 ==
  <OBJ_Abs_Long_Velocity> : Inport
  <OBJ_Abs_Long_Velocity_STD> : Inport  Port=2
  <OBJ_Abs_Lat_Velocity> : Inport  Port=3
  <OBJ_Abs_Lat_Velocity_STD> : Inport  Port=4
  Bus Creator : BusCreator  Inputs=4  OutDataTypeStr=Bus: FUS_VISION_OBJ_VELOCITY
      settings: InheritFromInputs=off
  Out1 : Outport
  wires:
  <OBJ_Abs_Lat_Velocity_STD>/1 -> Bus Creator/4
  <OBJ_Abs_Long_Velocity>/1 -> Bus Creator/1
  <OBJ_Abs_Lat_Velocity>/1 -> Bus Creator/3
  <OBJ_Abs_Long_Velocity_STD>/1 -> Bus Creator/2
  Bus Creator/1 -> Out1/1

== system fusionAlg/FUSION /FUS_DataAdapter/VisionAdapter/ObjAdapter/Obj_36/Subsystem2 ==
  <OBJ_Angle_Mid> : Inport
  <OBJ_Angle_Mid_STD> : Inport  Port=2
  Bus Creator : BusCreator  Inputs=2  OutDataTypeStr=Bus: FUS_VISION_OBJ_ANGLE_ST
      settings: InheritFromInputs=off
  Out1 : Outport
  wires:
  <OBJ_Angle_Mid>/1 -> Bus Creator/1
  Bus Creator/1 -> Out1/1
  <OBJ_Angle_Mid_STD>/1 -> Bus Creator/2

== system fusionAlg/FUSION /FUS_DataAdapter/VisionAdapter/ObjAdapter/Obj_36/Subsystem3 ==
  <OBJ_Abs_Long_Acc> : Inport
  <OBJ_Abs_Long_Acc_STD> : Inport  Port=2
  <OBJ_Abs_Lat_Acc> : Inport  Port=3
  <OBJ_Abs_Lat_Acc_STD> : Inport  Port=4
  Bus Creator : BusCreator  Inputs=4  OutDataTypeStr=Bus: FUS_VISION_OBJ_ACCE_ST
      settings: InheritFromInputs=off
  Out1 : Outport
  wires:
  <OBJ_Abs_Long_Acc_STD>/1 -> Bus Creator/2
  <OBJ_Abs_Long_Acc>/1 -> Bus Creator/1
  Bus Creator/1 -> Out1/1
  <OBJ_Abs_Lat_Acc_STD>/1 -> Bus Creator/4
  <OBJ_Abs_Lat_Acc>/1 -> Bus Creator/3

== system fusionAlg/FUSION /FUS_DataAdapter/VisionAdapter/ObjAdapter/Obj_36/Subsystem4 ==
  <OBJ_Length> : Inport
  <OBJ_Width> : Inport  Port=2
  <OBJ_Height> : Inport  Port=3
  Bus Creator : BusCreator  Inputs=3  OutDataTypeStr=Bus: FUS_VISION_BOXSIZE_ST
      settings: InheritFromInputs=off
  Out1 : Outport
  wires:
  Bus Creator/1 -> Out1/1
  <OBJ_Height>/1 -> Bus Creator/3
  <OBJ_Width>/1 -> Bus Creator/2
  <OBJ_Length>/1 -> Bus Creator/1

== system fusionAlg/FUSION /FUS_DataAdapter/VisionAdapter/ObjAdapter/Obj_36/Subsystem5 ==
  Bus Creator : BusCreator  Inputs=3  OutDataTypeStr=Bus: FUS_VISOBJ_UINT8_RESERVED_ST
      settings: InheritFromInputs=off
  Constant1 : Constant  Value=0  OutDataTypeStr=uint8
  Constant2 : Constant  Value=0  OutDataTypeStr=uint8
  Constant3 : Constant  Value=0  OutDataTypeStr=uint8
  reserved1 : Outport
  wires:
  Bus Creator/1 -> reserved1/1
  Constant2/1 -> Bus Creator/1
  Constant1/1 -> Bus Creator/2
  Constant3/1 -> Bus Creator/3

== system fusionAlg/FUSION /FUS_DataAdapter/VisionAdapter/ObjAdapter/Obj_36/Subsystem6 ==
  Bus Creator : BusCreator  Inputs=2  OutDataTypeStr=Bus: FUS_VISOBJ_UINT32_RESERVED_ST
      settings: InheritFromInputs=off
  Constant5 : Constant  Value=0  OutDataTypeStr=uint32
  Constant6 : Constant  Value=0  OutDataTypeStr=uint32
  reserved2 : Outport
  wires:
  Constant5/1 -> Bus Creator/1
  Bus Creator/1 -> reserved2/1
  Constant6/1 -> Bus Creator/2

== system fusionAlg/FUSION /FUS_DataAdapter/VisionAdapter/ObjAdapter/Obj_36/Subsystem7 ==
  note: Fusion
  note: 0 : (BIT_0)Old or New
  note: EyeQ4
  note: 1 : (BIT_1)Predicted or Measured
  note: 2 : (BIT_2)Not Valid or Valid
  note: 0 : Initialized
  note: 1 : Measured
  note: 2 : Predicted
  <OBJ_Measuring_Status> : Inport
  1-D Lookup Table : Lookup_n-D  NumberOfTableDimensions=1  BreakpointsForDimension1=[0,1,2,3,4,5,6,7]  IndexSearchMethod=Linear search  Table=[2,0,1,1,0,0,1,1]  InterpMethod=Flat  InternalRulePriority=Speed  RndMeth=Simplest  InputSameDT=on
  Data Type Conversion1 : DataTypeConversion  OutDataTypeStr=uint32
  Obj_Status : Outport
  wires:
  Data Type Conversion1/1 -> Obj_Status/1  "Obj_Status"
  <OBJ_Measuring_Status>/1 -> 1-D Lookup Table/1
  1-D Lookup Table/1 -> Data Type Conversion1/1  "Obj_Status"

== system fusionAlg/FUSION /FUS_DataAdapter/VisionAdapter/ObjAdapter/Obj_36/Subsystem8 ==
  note: 2 : Truck
  note: 1 : Pedestrian
  note: 2 : Vehicle
  note: 0 : Unfilled
  note: EyeQ4
  note: Fusion
  note: 0 : Unknown
  note: 1 : CAR
  note: 3 : Motorbike
  note: 4 : Bicycle
  note: 5 : Pedestrian
  note: 6 : General_Object
  note: 7 : Animal
  note: 8 : Uncertain_Vcl
  note: 3 : Truck
  note: 4: MoTor bike
  note: 5 : Bicycle
  note: 6 : General object
  note: 7 : Animal
  <OBJ_Object_Class> : Inport
  1-D Lookup Table : Lookup_n-D  NumberOfTableDimensions=1  BreakpointsForDimension1=[0,1,2,3,4,5,6,7,8]  IndexSearchMethod=Linear search  Table=[0,2,3,4,5,1,6,7,0]  InterpMethod=Flat  InternalRulePriority=Speed  RndMeth=Simplest  InputSameDT=on
  Data Type Conversion2 : DataTypeConversion  OutDataTypeStr=uint32
  Obj_Type : Outport
  wires:
  1-D Lookup Table/1 -> Data Type Conversion2/1  "Obj_Status"
  <OBJ_Object_Class>/1 -> 1-D Lookup Table/1
  Data Type Conversion2/1 -> Obj_Type/1  "Obj_Type"

== system fusionAlg/FUSION /FUS_DataAdapter/VisionAdapter/ObjAdapter/Obj_37/Obj_01_Agge ==
  <OBJ_Object_Age> : Inport
  Bus Creator : BusCreator  Inputs=4  OutDataTypeStr=Bus: FUS_VISION_OBJ_STAGE_AGE_ST
      settings: InheritFromInputs=off
  Constant : Constant  Value=3  OutDataTypeStr=uint16
  Constant1 : Constant  Value=2  OutDataTypeStr=uint16
  Data Type Conversion : DataTypeConversion  OutDataTypeStr=uint16
  Obj_01_Age : Outport  OutDataTypeStr=Bus: FUS_VISION_OBJ_STAGE_AGE_ST
  wires:
  Bus Creator/1 -> Obj_01_Age/1
  Constant/1 -> Bus Creator/2
  <OBJ_Object_Age>/1 -> Data Type Conversion/1
  Constant1/1 -> Bus Creator/4
  Data Type Conversion/1 -> Bus Creator/3, Bus Creator/1  "measureAge"

== system fusionAlg/FUSION /FUS_DataAdapter/VisionAdapter/ObjAdapter/Obj_37/Obj_01_boundarhy ==
  Bus Creator : BusCreator  Inputs=4  OutDataTypeStr=Bus: FUS_VISION_OBJ_BOUNDARY
      settings: InheritFromInputs=off
  Constant{,1..3} (4 alike) : Constant  Value=0  OutDataTypeStr=int16
  Obj_01_boundary : Outport  OutDataTypeStr=Bus: FUS_VISION_OBJ_BOUNDARY
  wires:
  Bus Creator/1 -> Obj_01_boundary/1
  Constant/1 -> Bus Creator/1
  Constant1/1 -> Bus Creator/2
  Constant2/1 -> Bus Creator/3
  Constant3/1 -> Bus Creator/4

== system fusionAlg/FUSION /FUS_DataAdapter/VisionAdapter/ObjAdapter/Obj_37/Subsystem ==
  <OBJ_Lat_Distance> : Inport
  <OBJ_Lat_Distance_STD> : Inport  Port=2
  <OBJ_Long_Distance> : Inport  Port=3
  <OBJ_Long_Distance_STD> : Inport  Port=4
  Bus Creator : BusCreator  Inputs=4  OutDataTypeStr=Bus: FUS_VISION_OBJ_COORD_ST
      settings: InheritFromInputs=off
  Obj_01_coordinate : Outport
  wires:
  <OBJ_Long_Distance>/1 -> Bus Creator/3
  <OBJ_Lat_Distance>/1 -> Bus Creator/1
  <OBJ_Lat_Distance_STD>/1 -> Bus Creator/2
  Bus Creator/1 -> Obj_01_coordinate/1
  <OBJ_Long_Distance_STD>/1 -> Bus Creator/4

== system fusionAlg/FUSION /FUS_DataAdapter/VisionAdapter/ObjAdapter/Obj_37/Subsystem1 ==
  <OBJ_Abs_Long_Velocity> : Inport
  <OBJ_Abs_Long_Velocity_STD> : Inport  Port=2
  <OBJ_Abs_Lat_Velocity> : Inport  Port=3
  <OBJ_Abs_Lat_Velocity_STD> : Inport  Port=4
  Bus Creator : BusCreator  Inputs=4  OutDataTypeStr=Bus: FUS_VISION_OBJ_VELOCITY
      settings: InheritFromInputs=off
  Out1 : Outport
  wires:
  <OBJ_Abs_Lat_Velocity_STD>/1 -> Bus Creator/4
  <OBJ_Abs_Long_Velocity>/1 -> Bus Creator/1
  <OBJ_Abs_Lat_Velocity>/1 -> Bus Creator/3
  <OBJ_Abs_Long_Velocity_STD>/1 -> Bus Creator/2
  Bus Creator/1 -> Out1/1

== system fusionAlg/FUSION /FUS_DataAdapter/VisionAdapter/ObjAdapter/Obj_37/Subsystem2 ==
  <OBJ_Angle_Mid> : Inport
  <OBJ_Angle_Mid_STD> : Inport  Port=2
  Bus Creator : BusCreator  Inputs=2  OutDataTypeStr=Bus: FUS_VISION_OBJ_ANGLE_ST
      settings: InheritFromInputs=off
  Out1 : Outport
  wires:
  <OBJ_Angle_Mid>/1 -> Bus Creator/1
  Bus Creator/1 -> Out1/1
  <OBJ_Angle_Mid_STD>/1 -> Bus Creator/2

== system fusionAlg/FUSION /FUS_DataAdapter/VisionAdapter/ObjAdapter/Obj_37/Subsystem3 ==
  <OBJ_Abs_Long_Acc> : Inport
  <OBJ_Abs_Long_Acc_STD> : Inport  Port=2
  <OBJ_Abs_Lat_Acc> : Inport  Port=3
  <OBJ_Abs_Lat_Acc_STD> : Inport  Port=4
  Bus Creator : BusCreator  Inputs=4  OutDataTypeStr=Bus: FUS_VISION_OBJ_ACCE_ST
      settings: InheritFromInputs=off
  Out1 : Outport
  wires:
  <OBJ_Abs_Long_Acc_STD>/1 -> Bus Creator/2
  <OBJ_Abs_Long_Acc>/1 -> Bus Creator/1
  Bus Creator/1 -> Out1/1
  <OBJ_Abs_Lat_Acc_STD>/1 -> Bus Creator/4
  <OBJ_Abs_Lat_Acc>/1 -> Bus Creator/3

== system fusionAlg/FUSION /FUS_DataAdapter/VisionAdapter/ObjAdapter/Obj_37/Subsystem4 ==
  <OBJ_Length> : Inport
  <OBJ_Width> : Inport  Port=2
  <OBJ_Height> : Inport  Port=3
  Bus Creator : BusCreator  Inputs=3  OutDataTypeStr=Bus: FUS_VISION_BOXSIZE_ST
      settings: InheritFromInputs=off
  Out1 : Outport
  wires:
  Bus Creator/1 -> Out1/1
  <OBJ_Height>/1 -> Bus Creator/3
  <OBJ_Width>/1 -> Bus Creator/2
  <OBJ_Length>/1 -> Bus Creator/1

== system fusionAlg/FUSION /FUS_DataAdapter/VisionAdapter/ObjAdapter/Obj_37/Subsystem5 ==
  Bus Creator : BusCreator  Inputs=3  OutDataTypeStr=Bus: FUS_VISOBJ_UINT8_RESERVED_ST
      settings: InheritFromInputs=off
  Constant1 : Constant  Value=0  OutDataTypeStr=uint8
  Constant2 : Constant  Value=0  OutDataTypeStr=uint8
  Constant3 : Constant  Value=0  OutDataTypeStr=uint8
  reserved1 : Outport
  wires:
  Bus Creator/1 -> reserved1/1
  Constant2/1 -> Bus Creator/1
  Constant1/1 -> Bus Creator/2
  Constant3/1 -> Bus Creator/3

== system fusionAlg/FUSION /FUS_DataAdapter/VisionAdapter/ObjAdapter/Obj_37/Subsystem6 ==
  Bus Creator : BusCreator  Inputs=2  OutDataTypeStr=Bus: FUS_VISOBJ_UINT32_RESERVED_ST
      settings: InheritFromInputs=off
  Constant5 : Constant  Value=0  OutDataTypeStr=uint32
  Constant6 : Constant  Value=0  OutDataTypeStr=uint32
  reserved2 : Outport
  wires:
  Constant5/1 -> Bus Creator/1
  Bus Creator/1 -> reserved2/1
  Constant6/1 -> Bus Creator/2

== system fusionAlg/FUSION /FUS_DataAdapter/VisionAdapter/ObjAdapter/Obj_37/Subsystem7 ==
  note: Fusion
  note: 0 : (BIT_0)Old or New
  note: EyeQ4
  note: 1 : (BIT_1)Predicted or Measured
  note: 2 : (BIT_2)Not Valid or Valid
  note: 0 : Initialized
  note: 1 : Measured
  note: 2 : Predicted
  <OBJ_Measuring_Status> : Inport
  1-D Lookup Table : Lookup_n-D  NumberOfTableDimensions=1  BreakpointsForDimension1=[0,1,2,3,4,5,6,7]  IndexSearchMethod=Linear search  Table=[2,0,1,1,0,0,1,1]  InterpMethod=Flat  InternalRulePriority=Speed  RndMeth=Simplest  InputSameDT=on
  Data Type Conversion1 : DataTypeConversion  OutDataTypeStr=uint32
  Obj_Status : Outport
  wires:
  Data Type Conversion1/1 -> Obj_Status/1  "Obj_Status"
  <OBJ_Measuring_Status>/1 -> 1-D Lookup Table/1
  1-D Lookup Table/1 -> Data Type Conversion1/1  "Obj_Status"

== system fusionAlg/FUSION /FUS_DataAdapter/VisionAdapter/ObjAdapter/Obj_37/Subsystem8 ==
  note: 2 : Truck
  note: 1 : Pedestrian
  note: 2 : Vehicle
  note: 0 : Unfilled
  note: EyeQ4
  note: Fusion
  note: 0 : Unknown
  note: 1 : CAR
  note: 3 : Motorbike
  note: 4 : Bicycle
  note: 5 : Pedestrian
  note: 6 : General_Object
  note: 7 : Animal
  note: 8 : Uncertain_Vcl
  note: 3 : Truck
  note: 4: MoTor bike
  note: 5 : Bicycle
  note: 6 : General object
  note: 7 : Animal
  <OBJ_Object_Class> : Inport
  1-D Lookup Table : Lookup_n-D  NumberOfTableDimensions=1  BreakpointsForDimension1=[0,1,2,3,4,5,6,7,8]  IndexSearchMethod=Linear search  Table=[0,2,3,4,5,1,6,7,0]  InterpMethod=Flat  InternalRulePriority=Speed  RndMeth=Simplest  InputSameDT=on
  Data Type Conversion2 : DataTypeConversion  OutDataTypeStr=uint32
  Obj_Type : Outport
  wires:
  1-D Lookup Table/1 -> Data Type Conversion2/1  "Obj_Status"
  <OBJ_Object_Class>/1 -> 1-D Lookup Table/1
  Data Type Conversion2/1 -> Obj_Type/1  "Obj_Type"

== system fusionAlg/FUSION /FUS_DataAdapter/VisionAdapter/ObjAdapter/Obj_38/Obj_01_Agge ==
  <OBJ_Object_Age> : Inport
  Bus Creator : BusCreator  Inputs=4  OutDataTypeStr=Bus: FUS_VISION_OBJ_STAGE_AGE_ST
      settings: InheritFromInputs=off
  Constant : Constant  Value=3  OutDataTypeStr=uint16
  Constant1 : Constant  Value=2  OutDataTypeStr=uint16
  Data Type Conversion : DataTypeConversion  OutDataTypeStr=uint16
  Obj_01_Age : Outport  OutDataTypeStr=Bus: FUS_VISION_OBJ_STAGE_AGE_ST
  wires:
  Bus Creator/1 -> Obj_01_Age/1
  Constant/1 -> Bus Creator/2
  <OBJ_Object_Age>/1 -> Data Type Conversion/1
  Constant1/1 -> Bus Creator/4
  Data Type Conversion/1 -> Bus Creator/3, Bus Creator/1  "measureAge"

== system fusionAlg/FUSION /FUS_DataAdapter/VisionAdapter/ObjAdapter/Obj_38/Obj_01_boundarhy ==
  Bus Creator : BusCreator  Inputs=4  OutDataTypeStr=Bus: FUS_VISION_OBJ_BOUNDARY
      settings: InheritFromInputs=off
  Constant{,1..3} (4 alike) : Constant  Value=0  OutDataTypeStr=int16
  Obj_01_boundary : Outport  OutDataTypeStr=Bus: FUS_VISION_OBJ_BOUNDARY
  wires:
  Bus Creator/1 -> Obj_01_boundary/1
  Constant/1 -> Bus Creator/1
  Constant1/1 -> Bus Creator/2
  Constant2/1 -> Bus Creator/3
  Constant3/1 -> Bus Creator/4

== system fusionAlg/FUSION /FUS_DataAdapter/VisionAdapter/ObjAdapter/Obj_38/Subsystem ==
  <OBJ_Lat_Distance> : Inport
  <OBJ_Lat_Distance_STD> : Inport  Port=2
  <OBJ_Long_Distance> : Inport  Port=3
  <OBJ_Long_Distance_STD> : Inport  Port=4
  Bus Creator : BusCreator  Inputs=4  OutDataTypeStr=Bus: FUS_VISION_OBJ_COORD_ST
      settings: InheritFromInputs=off
  Obj_01_coordinate : Outport
  wires:
  <OBJ_Long_Distance>/1 -> Bus Creator/3
  <OBJ_Lat_Distance>/1 -> Bus Creator/1
  <OBJ_Lat_Distance_STD>/1 -> Bus Creator/2
  Bus Creator/1 -> Obj_01_coordinate/1
  <OBJ_Long_Distance_STD>/1 -> Bus Creator/4

== system fusionAlg/FUSION /FUS_DataAdapter/VisionAdapter/ObjAdapter/Obj_38/Subsystem1 ==
  <OBJ_Abs_Long_Velocity> : Inport
  <OBJ_Abs_Long_Velocity_STD> : Inport  Port=2
  <OBJ_Abs_Lat_Velocity> : Inport  Port=3
  <OBJ_Abs_Lat_Velocity_STD> : Inport  Port=4
  Bus Creator : BusCreator  Inputs=4  OutDataTypeStr=Bus: FUS_VISION_OBJ_VELOCITY
      settings: InheritFromInputs=off
  Out1 : Outport
  wires:
  <OBJ_Abs_Lat_Velocity_STD>/1 -> Bus Creator/4
  <OBJ_Abs_Long_Velocity>/1 -> Bus Creator/1
  <OBJ_Abs_Lat_Velocity>/1 -> Bus Creator/3
  <OBJ_Abs_Long_Velocity_STD>/1 -> Bus Creator/2
  Bus Creator/1 -> Out1/1

== system fusionAlg/FUSION /FUS_DataAdapter/VisionAdapter/ObjAdapter/Obj_38/Subsystem2 ==
  <OBJ_Angle_Mid> : Inport
  <OBJ_Angle_Mid_STD> : Inport  Port=2
  Bus Creator : BusCreator  Inputs=2  OutDataTypeStr=Bus: FUS_VISION_OBJ_ANGLE_ST
      settings: InheritFromInputs=off
  Out1 : Outport
  wires:
  <OBJ_Angle_Mid>/1 -> Bus Creator/1
  Bus Creator/1 -> Out1/1
  <OBJ_Angle_Mid_STD>/1 -> Bus Creator/2

== system fusionAlg/FUSION /FUS_DataAdapter/VisionAdapter/ObjAdapter/Obj_38/Subsystem3 ==
  <OBJ_Abs_Long_Acc> : Inport
  <OBJ_Abs_Long_Acc_STD> : Inport  Port=2
  <OBJ_Abs_Lat_Acc> : Inport  Port=3
  <OBJ_Abs_Lat_Acc_STD> : Inport  Port=4
  Bus Creator : BusCreator  Inputs=4  OutDataTypeStr=Bus: FUS_VISION_OBJ_ACCE_ST
      settings: InheritFromInputs=off
  Out1 : Outport
  wires:
  <OBJ_Abs_Long_Acc_STD>/1 -> Bus Creator/2
  <OBJ_Abs_Long_Acc>/1 -> Bus Creator/1
  Bus Creator/1 -> Out1/1
  <OBJ_Abs_Lat_Acc_STD>/1 -> Bus Creator/4
  <OBJ_Abs_Lat_Acc>/1 -> Bus Creator/3
